simulink model "FullBridgeInverter"  (R2023b)
settings: Solver=VariableStepAuto  StartTime=0.0  StopTime=0.01  RelTol=1e-3
libraries: spsDiodeLib x4, spsMosfetLib x4, spsSeriesRLCBranchLib x3, spsCurrentMeasurementLib x2, spsDCVoltageSourceLib x1, spsVoltageMeasurementLib x1, sps_lib x1
settings Model: Creator=yagiz  LastModifiedBy=yagiz

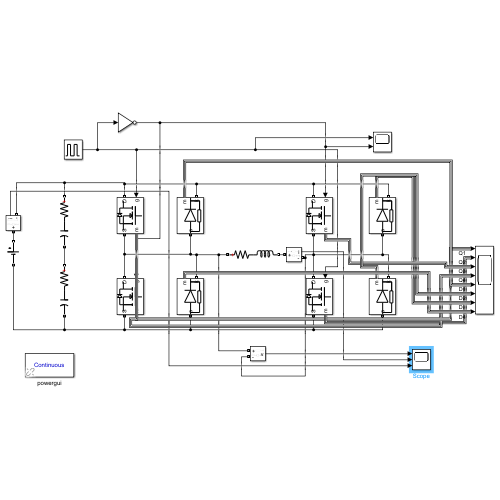
[thumbnail: Simulink's stored preview of the top-level diagram]
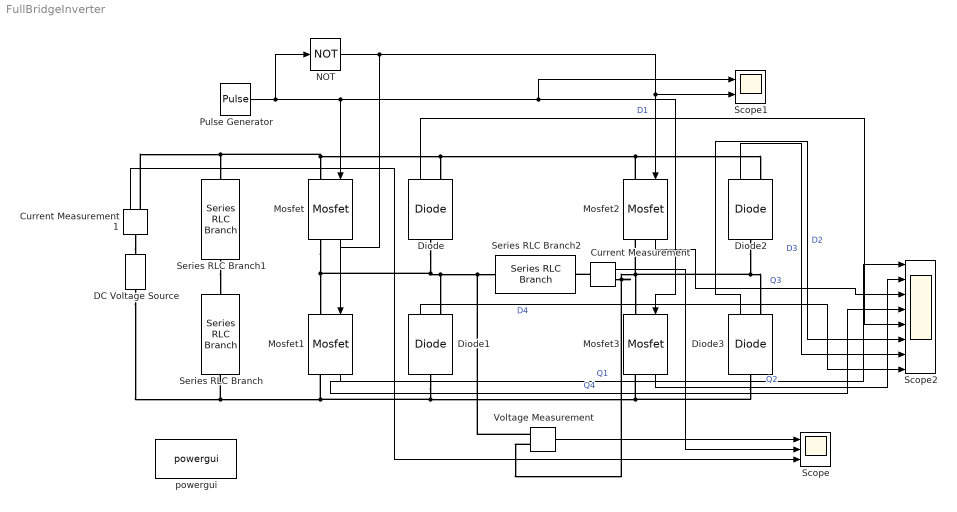
== system FullBridgeInverter ==
  Current Measurement : spsCurrentMeasurementLib/Current Measurement  PhasorSimulation=off  OutputType=Complex  PSBequivalent=0
  Current Measurement1 : spsCurrentMeasurementLib/Current Measurement  PhasorSimulation=off  OutputType=Complex  PSBequivalent=0
  DC Voltage Source : spsDCVoltageSourceLib/DC Voltage Source  Amplitude=50  Measurements=None
  Diode{,1..3} (4 alike) : spsDiodeLib/Diode  Ron=0.001  Lon=0  Vf=0  IC=0  UseSnubber=0  Rs=500  Cs=250e-9  Measurements=on
  Mosfet{,1..3} (4 alike) : spsMosfetLib/Mosfet  Ron=0.1  Lon=0  Rd=0.01  Vfd=0  IC=0  Rs=1e5  Cs=inf  Measurements=on
  NOT : Logic  Operator=NOT  IconShape=distinctive  AllPortsSameDT=off  OutDataTypeStr=boolean
  Pulse Generator : DiscretePulseGenerator  PulseType=Time based  Period=1/40000  PulseWidth=50
  Scope : Scope  NumInputPorts=3
  Scope1 : Scope  NumInputPorts=2
  Scope2 : Scope  NumInputPorts=8
  Series RLC Branch : spsSeriesRLCBranchLib/Series RLC Branch  LConnTagsString=__new0  RConnTagsString=__new0  BranchType=RC  Resistance=0.001  Inductance=1e-3  SetiL0=off  InitialCurrent=0  Capacitance=1  Setx0=off  InitialVoltage=0  Measurements=None
  Series RLC Branch1 : spsSeriesRLCBranchLib/Series RLC Branch  LConnTagsString=__new0  RConnTagsString=__new0  BranchType=RC  Resistance=0.001  Inductance=1e-3  SetiL0=off  InitialCurrent=0  Capacitance=1  Setx0=off  InitialVoltage=0  Measurements=None
  Series RLC Branch2 : spsSeriesRLCBranchLib/Series RLC Branch  LConnTagsString=__new0  RConnTagsString=__new0  BranchType=RL  Resistance=10  Inductance=1e-4  SetiL0=off  InitialCurrent=0  Capacitance=1e-6  Setx0=off  InitialVoltage=0  Measurements=None
  Voltage Measurement : spsVoltageMeasurementLib/Voltage Measurement  PhasorSimulation=off  OutputType=Complex  PSBequivalent=0
  powergui : sps_lib/powergui  Priority=1  SimulationMode=Continuous  SampleTime=50e-6  frequency=60  Iterations=50  frequencyindice=0  Pbase=100e6  ErrMax=1e-4  UnitsV=kV  UnitsW=MW  buscounter=0  FunctionMessages=off  echomessages=off  EnableUseOfTLC=off  CurrentSourceSwitches=off  DisableSnubberDevices=off  DisableRonSwitches=off  DisableVfSwitches=off  DisplayEquations=off  AutomaticDiscreteSolvers=off  SolverType=Tustin/Backward Euler (TBE)  Interpol=off  ExternalGateDelay=off  methode=off  Ts=100  x0status=blocks  SPID=on  SwTol=0  HookPort=off  NonlinearTolerance=1e-4  nMaxIteration=100  ContinueOnMaxIteration=off  RestoreLinks=warning  ResistiveCurrentMeasurement=off  Frange=[0:2:500]  Ylog=off  Xlog=on  ShowGrid=off  save=off  variable=ZData  structure=0  ZoomFFT=off  StartTime=0.0  cycles=1  DisplayStyle=1  fundamental=60  FreqAxis=off  MaxFrequency=1000  frequencyindicesteady=1  RmsSteady=1  display=off
  wires:
  Pulse Generator/1 -> NOT/1, Mosfet/1, Mosfet3/1, Scope1/1
  NOT/1 -> Mosfet2/1, Scope1/2, Mosfet1/1
  Current Measurement/1 -> Scope/2
  Voltage Measurement/1 -> Scope/1
  Mosfet/1 -> Scope2/1  "Q1"
  Mosfet1/1 -> Scope2/4  "Q4"
  Mosfet3/1 -> Scope2/2  "Q2"
  Diode1/1 -> Scope2/8  "D4"
  Diode/1 -> Scope2/5  "D1"
  Diode2/1 -> Scope2/7  "D3"
  Diode3/1 -> Scope2/6  "D2"
  Mosfet2/1 -> Scope2/3  "Q3"
  Current Measurement1/1 -> Scope/3
  connections:
  Series RLC Branch1/RConn1 -- Series RLC Branch/LConn1
  Diode/LConn1 -- Mosfet/RConn1 -- Mosfet1/LConn1 -- Voltage Measurement/LConn1 -- Series RLC Branch2/LConn1 -- Diode1/RConn1
  Diode2/LConn1 -- Diode3/RConn1 -- Mosfet2/RConn1 -- Mosfet3/LConn1 -- Voltage Measurement/LConn2 -- Current Measurement/RConn1
  Mosfet2/LConn1 -- Diode2/RConn1 -- Diode/RConn1 -- Mosfet/LConn1 -- Current Measurement1/RConn1 -- Series RLC Branch1/LConn1
  DC Voltage Source/LConn1 -- Diode1/LConn1 -- Diode3/LConn1 -- Mosfet3/RConn1 -- Mosfet1/RConn1 -- Series RLC Branch/RConn1
  Current Measurement/LConn1 -- Series RLC Branch2/RConn1
  Current Measurement1/LConn1 -- DC Voltage Source/RConn1
